simulink model "naibaoOSTBC_22"  (R2018a)
settings: Solver=FixedStepDiscrete  StartTime=0.0  StopTime=10  RelTol=1e-3
model workspace (MAT data in the model file):
  FrameLen = 100
  SampleTime = 0.001
  maxNumBits = 100000000
  maxNumErrs = 1000
libraries: commdigbbndpm3 x2, commchan3 x1, commrandsrc3 x1, commsink2 x1, commmimo x1
settings Model: Creator=myste  LastModifiedBy=myste
settings DataIOCC: SaveOutput=off  SaveTime=off

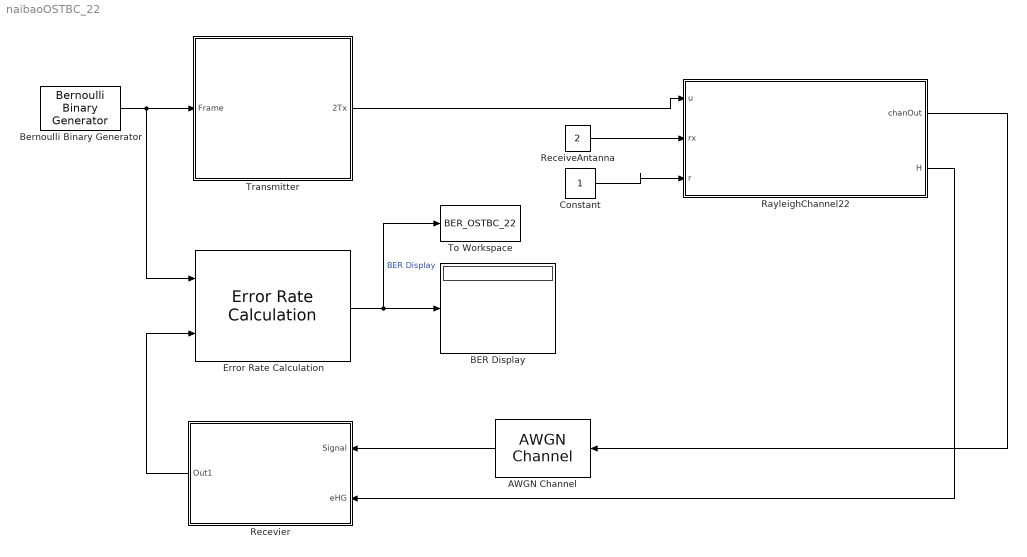
== system naibaoOSTBC_22 ==
  AWGN Channel : commchan3/AWGN Channel  InputProcessing=Columns as channels (frame based)  seed=67  noiseMode="Signal to noise ratio  (Eb/No)"  EbNodB=EbNo  EsNodB=2  SNRdB=10  bitsPerSym=1  Ps=1  Tsym=SampleTime  variance=1
  BER Display : Display
  Bernoulli Binary Generator : commrandsrc3/Bernoulli Binary Generator  ProbabilityOfZero=0.5  SeedSource=Auto  Seed=61  SampleTime=SampleTime  SamplesPerFrame=FrameLen  OutputDataType=boolean  SimulateUsing=Interpreted execution
  Constant : Constant
  Error Rate Calculation : commsink2/Error Rate Calculation  N=0  st_delay=0  cp_mode=Entire frame  subframe=[]  PMode=Port  WsName=ErrorVec  RsMode2=off  stop=on  numErr=maxNumErrs  maxBits=maxNumBits
  RayleighChannel22 : MATLAB Function  TreatAsAtomicUnit=on
  ReceiveAntanna : Constant  Value=2
  Recevier : Subsystem
  To Workspace : ToWorkspace  VariableName=BER_OSTBC_22  SampleTime=-1
      settings: MaxDataPoints=1  Save2DSignal=2-D array (concatenate along first dimension)
  Transmitter : Subsystem
  wires:
  Bernoulli Binary Generator/1 -> Error Rate Calculation/1, Transmitter/1(Frame)
  AWGN Channel/1 -> Recevier/1(Signal)
  Recevier/1(Out1) -> Error Rate Calculation/2
  Error Rate Calculation/1 -> To Workspace/1, BER Display/1  "BER Display"
  ReceiveAntanna/1 -> RayleighChannel22/2(rx)
  RayleighChannel22/1(chanOut) -> AWGN Channel/1
  RayleighChannel22/2(H) -> Recevier/2(eHG)
  Transmitter/1(2Tx) -> RayleighChannel22/1(u)
  Constant/1 -> RayleighChannel22/3(r)

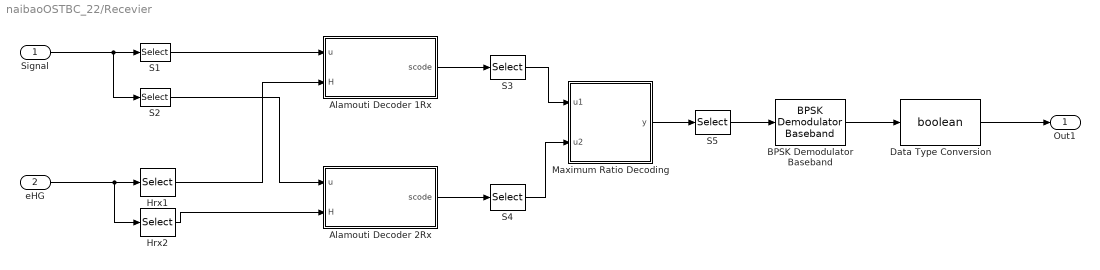
== system naibaoOSTBC_22/Recevier ==
  Signal : Inport
  eHG : Inport  Port=2
  Alamouti Decoder 1Rx : MATLAB Function  TreatAsAtomicUnit=on
  Alamouti Decoder 2Rx : MATLAB Function  TreatAsAtomicUnit=on
  BPSK Demodulator Baseband : commdigbbndpm3/BPSK Demodulator Baseband  DecType=Hard decision  VarSource=Dialog  Variance=1  Ph=0  outDtype=Inherit via internal rule  derotateFactorWordLen=16  derotateFactorDataTypeStr=Inherit: Same word length as input  derotateFactorLastDataTypeStr=Inherit: Same word length as input
  Data Type Conversion : DataTypeConversion  OutDataTypeStr=boolean
  Hrx1 : Selector  NumberOfDimensions=3  InputPortWidth=3  IndexOptions=Select all,Select all,Index vector (dialog)  Indices=[1 3],1,1  OutputSizes=1,1,1
  Hrx2 : Selector  NumberOfDimensions=3  InputPortWidth=3  IndexOptions=Select all,Select all,Index vector (dialog)  Indices=[1 3],1,2  OutputSizes=1,1,1
  Maximum Ratio Decoding : MATLAB Function  TreatAsAtomicUnit=on
  S{1,3..5} (4 alike) : Selector  NumberOfDimensions=2  InputPortWidth=3  IndexOptions=Select all,Index vector (dialog)  Indices=[1 3],1  OutputSizes=1,1
  S2 : Selector  NumberOfDimensions=2  InputPortWidth=3  IndexOptions=Select all,Index vector (dialog)  Indices=[1 3],2  OutputSizes=1,1
  Out1 : Outport
  wires:
  eHG/1 -> Hrx2/1, Hrx1/1
  Signal/1 -> S2/1, S1/1
  S1/1 -> Alamouti Decoder 1Rx/1(u)
  Hrx2/1 -> Alamouti Decoder 2Rx/2(H)
  Alamouti Decoder 1Rx/1(scode) -> S3/1
  Alamouti Decoder 2Rx/1(scode) -> S4/1
  S3/1 -> Maximum Ratio Decoding/1(u1)
  S4/1 -> Maximum Ratio Decoding/2(u2)
  Maximum Ratio Decoding/1(y) -> S5/1
  Hrx1/1 -> Alamouti Decoder 1Rx/2(H)
  S2/1 -> Alamouti Decoder 2Rx/1(u)
  S5/1 -> BPSK Demodulator Baseband/1
  Data Type Conversion/1 -> Out1/1
  BPSK Demodulator Baseband/1 -> Data Type Conversion/1

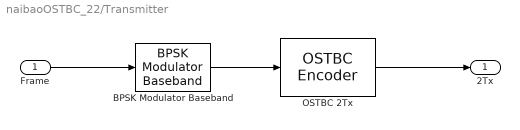
== system naibaoOSTBC_22/Transmitter ==
  Frame : Inport
  BPSK Modulator Baseband : commdigbbndpm3/BPSK Modulator Baseband  Ph=0  outDtype=double  outWordLen=16  outUDDataType=sfix(16)  outFracLenMode=Best precision  outFracLen=15  outDataTypeStr=double  outLastDataTypeStr=double
  OSTBC 2Tx : commmimo/OSTBC Encoder  numTx=2  rate=3/4  overflowMode=Wrap  OvFlMode=off  OvFlModeLastStrValue=off
      settings: SourceProductName=Communications System Toolbox  SourceProductBaseCode=CM
  2Tx : Outport
  wires:
  Frame/1 -> BPSK Modulator Baseband/1
  OSTBC 2Tx/1 -> 2Tx/1
  BPSK Modulator Baseband/1 -> OSTBC 2Tx/1

== matlab function naibaoOSTBC_22/Recevier/Alamouti Decoder 1Rx ==
  data: u input; scode output; H input
function scode= AlamoutiDecoder(u,H)
%% 基本参数
s=size(u);
%得到帧长
FrameLength=s(1);
%输出序列
scode=complex(zeros(FrameLength,2));
for i = 1:FrameLength/2
    scode(2*i-1,1) = H(2*i,1)' *  u(2*i-1) + H(2*i,2) * u(2*i)';
    scode(2*i,1) = H(2*i,2)' *  u(2*i-1) - H(2*i,1) * u(2*i)';
end

== matlab function naibaoOSTBC_22/RayleighChannel22 ==
  data: u input; chanOut output; H output; rx input; r input
function [chanOut,H] = RayleighChannel22(u,rx,r)
%得到Rayleigh信道，u为发射天线的信息，rx为接收天线的个数,r为编码速率
%% 初始化参数
% 获取输入帧长,输入天线数
s=size(u);
FrameLength=s(1);
N=s(2);
%接收天线数
M=rx;
%两个时隙中信道参数保持不变
Num=0;
%生成信道矩阵
H = complex( zeros(FrameLength, N, 2) );
%% 生成信道并计算输出
%计算Num
if s(2)==2 
    Num=4;
end
if s(2)==4 && r==3/4
    Num=8;
end
if s(2)==4 && r==1/2
    Num=16;
end
%生成分组中，第一个分组中的信道增益
H(1:Num:end, :, :) = (randn(FrameLength/Num, N, M) + ...
                         1i*randn(FrameLength/Num, N, 2))/sqrt(2);
%assume held constant for other symbol periods
for i=2:Num
    H(i:Num:end, :, :) = H(1:Num:end, :, :);
end
%第一个接收天线的信道矩阵
H21 = H(:,:,1)/sqrt(2);
%第二个接收天线的信道矩阵
H22 = H(:,:,2)/sqrt(2);
%输出接收天线1信号
chanOut21 = sum(H21.* u, 2);
%输出接收天线2信号
chanOut22 = sum(H22.* u, 2);
%输出信号
chanOut=[chanOut21,chanOut22];

== matlab function naibaoOSTBC_22/Recevier/Alamouti Decoder 2Rx ==
  data: u input; scode output; H input
function scode = AlamoutiDecoder(u,H)
%% 基本参数
s=size(u);
%得到帧长
FrameLength=s(1);
%输出序列
scode=complex(zeros(FrameLength,2));
for i = 1:FrameLength/2
    scode(2*i-1,1) = H(2*i,1)' *  u(2*i-1) + H(2*i,2) * u(2*i)';
    scode(2*i,1) = H(2*i,2)' *  u(2*i-1) - H(2*i,1) * u(2*i)';;
end

== matlab function naibaoOSTBC_22/Recevier/Maximum Ratio Decoding ==
  data: u1 input; y output; u2 input
function y = mrd(u1,u2)
%两条信道完全对称,直接等增益合并
s=size(u1);
y=complex( zeros(s(1),2));
for i=1:s(1)
    y(i,1)=(u1(i)+u2(i))/2;
end
